simulink model "AC_DC_Converter"  (R2024a)
settings: Solver=VariableStepAuto  StartTime=0.0  StopTime=0.02  RelTol=1e-3
libraries: spsDiodeLib x5, spsSeriesRLCBranchLib x5, spsVoltageMeasurementLib x3, spsACVoltageSourceLib x1, spsLinearTransformerLib x1, spsMosfetLib x1, sps_lib x1
settings Model: Creator=Ketan  LastModifiedBy=Ketan

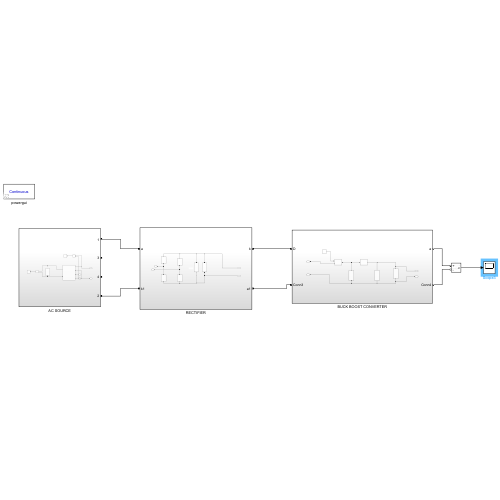
[thumbnail: Simulink's stored preview of the top-level diagram]
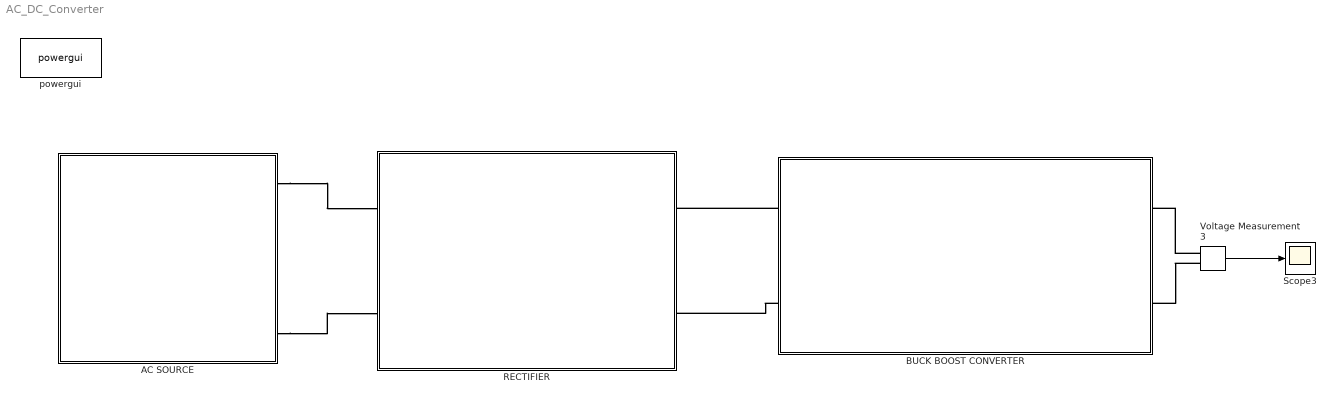
== system AC_DC_Converter ==
  AC SOURCE : Subsystem
  BUCK BOOST CONVERTER : Subsystem
  RECTIFIER : Subsystem
  Scope3 : Scope
  Voltage Measurement3 : spsVoltageMeasurementLib/Voltage Measurement  PhasorSimulation=off  OutputType=Complex  PSBequivalent=0
  powergui : sps_lib/powergui  Priority=1  SimulationMode=Continuous  SampleTime=50e-6  frequency=60  Iterations=50  frequencyindice=50  Pbase=100e6  ErrMax=1e-4  UnitsV=kV  UnitsW=MW  buscounter=0  FunctionMessages=off  echomessages=off  EnableUseOfTLC=off  CurrentSourceSwitches=off  DisableSnubberDevices=off  DisableRonSwitches=off  DisableVfSwitches=off  DisplayEquations=off  AutomaticDiscreteSolvers=off  SolverType=Tustin/Backward Euler (TBE)  Interpol=off  ExternalGateDelay=off  methode=off  Ts=100  x0status=blocks  SPID=on  SwTol=0  HookPort=off  NonlinearTolerance=1e-4  nMaxIteration=100  ContinueOnMaxIteration=off  RestoreLinks=warning  ResistiveCurrentMeasurement=off  Frange=[0:2:500]  Ylog=off  Xlog=on  ShowGrid=off  save=off  variable=ZData  structure=0  ZoomFFT=off  StartTime=0.0  cycles=1  DisplayStyle=1  fundamental=60  FreqAxis=off  MaxFrequency=1000  frequencyindicesteady=1  RmsSteady=1  display=off
  wires:
  Voltage Measurement3/1 -> Scope3/1
  connections:
  BUCK BOOST CONVERTER/LConn1 -- RECTIFIER/RConn1
  Voltage Measurement3/LConn1 -- BUCK BOOST CONVERTER/RConn1
  BUCK BOOST CONVERTER/LConn2 -- RECTIFIER/RConn2
  Voltage Measurement3/LConn2 -- BUCK BOOST CONVERTER/RConn2
  AC SOURCE/RConn1 -- RECTIFIER/LConn1
  AC SOURCE/RConn4 -- RECTIFIER/LConn2

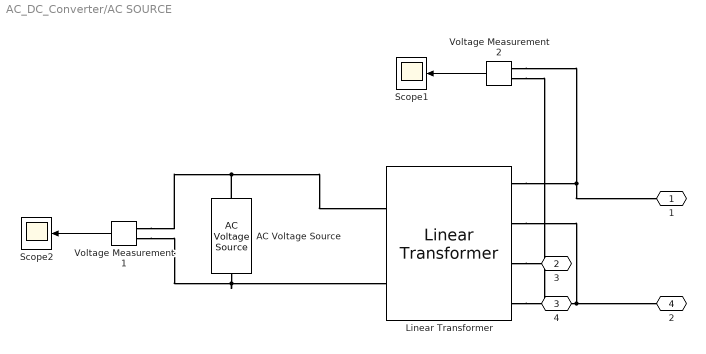
== system AC_DC_Converter/AC SOURCE ==
  AC Voltage Source : spsACVoltageSourceLib/AC Voltage Source  Amplitude=220*sqrt(2)  Phase=0  Frequency=50  SampleTime=0  Measurements=None  BusType=swing  Pref=10e3  Qref=0  Qmin=-inf  Qmax=+inf
  Linear Transformer : spsLinearTransformerLib/Linear Transformer  UNITS=pu  NominalPower=[ 250e6 60 ]  winding1="[ 220  0.002  0.08 ]"  winding2="[ 110  0.002  0.08 ]"  ThreeWindings=on  winding3=[ 110 0.002 0.08 ]  RmLm=[ 500 500 ]  Measurements=None  DataType=off
  Scope1 : Scope
  Scope2 : Scope
  Voltage Measurement1 : spsVoltageMeasurementLib/Voltage Measurement  PhasorSimulation=off  OutputType=Complex  PSBequivalent=0
  Voltage Measurement2 : spsVoltageMeasurementLib/Voltage Measurement  PhasorSimulation=off  OutputType=Complex  PSBequivalent=0
  1 : PMIOPort  Side=Right
  3 : PMIOPort  Port=2  Side=Right
  4 : PMIOPort  Port=3  Side=Right
  2 : PMIOPort  Port=4  Side=Right
  wires:
  Voltage Measurement1/1 -> Scope2/1
  Voltage Measurement2/1 -> Scope1/1
  connections:
  AC Voltage Source/RConn1 -- Linear Transformer/LConn1 -- Voltage Measurement1/LConn1
  AC Voltage Source/LConn1 -- Linear Transformer/LConn2 -- Voltage Measurement1/LConn2
  Voltage Measurement2/LConn2 -- 2/RConn1 -- Linear Transformer/RConn2
  Voltage Measurement2/LConn1 -- 1/RConn1 -- Linear Transformer/RConn1
  Linear Transformer/RConn4 -- 4/RConn1
  Linear Transformer/RConn3 -- 3/RConn1

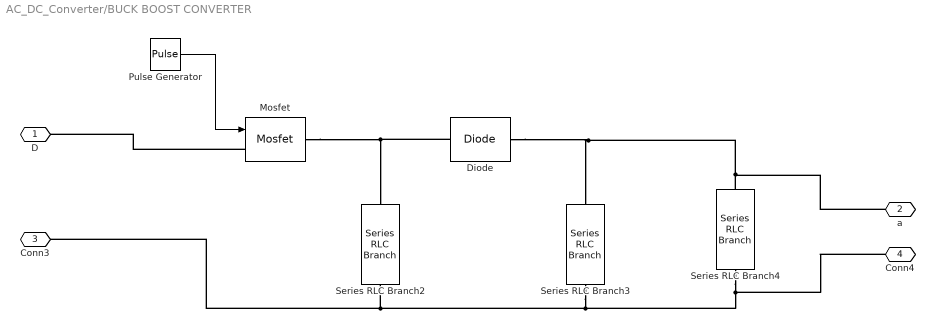
== system AC_DC_Converter/BUCK BOOST CONVERTER ==
  Diode : spsDiodeLib/Diode  Ron=0.001  Lon=0  Vf=0.8  IC=0  UseSnubber=0  Rs=500  Cs=250e-9  Measurements=off
  Mosfet : spsMosfetLib/Mosfet  Ron=0.1  Lon=0  Rd=0.01  Vfd=0  IC=0  Rs=1e5  Cs=inf  Measurements=off
  Pulse Generator : DiscretePulseGenerator  PulseType=Time based  Period=1/40000  PulseWidth=0.536*100
  Series RLC Branch2 : spsSeriesRLCBranchLib/Series RLC Branch  LConnTagsString=__new0  RConnTagsString=__new0  BranchType=L  Resistance=1  Inductance=45e-6  SetiL0=off  InitialCurrent=0  Capacitance=1e-6  Setx0=off  InitialVoltage=0  Measurements=None
  Series RLC Branch3 : spsSeriesRLCBranchLib/Series RLC Branch  LConnTagsString=__new0  RConnTagsString=__new0  BranchType=C  Resistance=1  Inductance=1e-3  SetiL0=off  InitialCurrent=0  Capacitance=8.5e-6  Setx0=off  InitialVoltage=0  Measurements=None
  Series RLC Branch4 : spsSeriesRLCBranchLib/Series RLC Branch  LConnTagsString=__new0  RConnTagsString=__new0  BranchType=R  Resistance=10  Inductance=1e-3  SetiL0=off  InitialCurrent=0  Capacitance=1e-6  Setx0=off  InitialVoltage=0  Measurements=None
  D : PMIOPort  Side=Left
  a : PMIOPort  Port=2  Side=Right
  Conn3 : PMIOPort  Port=3  Side=Left
  Conn4 : PMIOPort  Port=4  Side=Right
  wires:
  Pulse Generator/1 -> Mosfet/1
  connections:
  Mosfet/RConn1 -- Diode/RConn1 -- Series RLC Branch2/LConn1
  Series RLC Branch4/LConn1 -- Diode/LConn1 -- Series RLC Branch3/LConn1 -- a/RConn1
  Mosfet/LConn1 -- D/RConn1
  Series RLC Branch4/RConn1 -- Conn4/RConn1 -- Series RLC Branch3/RConn1 -- Conn3/RConn1 -- Series RLC Branch2/RConn1

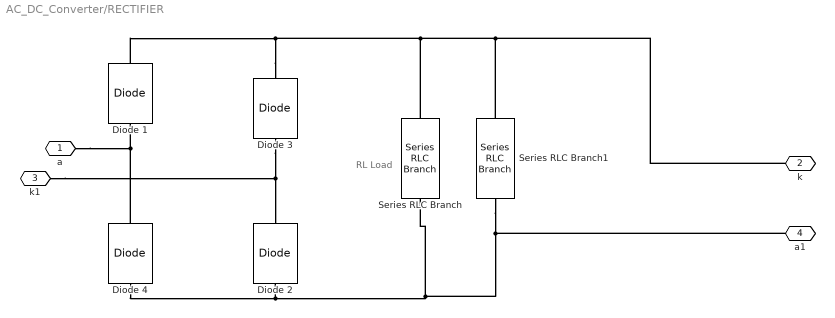
== system AC_DC_Converter/RECTIFIER ==
  note: RL Load
  Diode {1..4} (4 alike) : spsDiodeLib/Diode  Ron=0.001  Lon=0  Vf=0.8  IC=0  UseSnubber=0  Rs=500  Cs=250e-9  Measurements=off
  Series RLC Branch : spsSeriesRLCBranchLib/Series RLC Branch  LConnTagsString=__new0  RConnTagsString=__new0  BranchType=RL  Resistance=1  Inductance=1e-1  SetiL0=off  InitialCurrent=0  Capacitance=0  Setx0=off  InitialVoltage=0  Measurements=None
  Series RLC Branch1 : spsSeriesRLCBranchLib/Series RLC Branch  LConnTagsString=__new0  RConnTagsString=__new0  BranchType=C  Resistance=1  Inductance=1e-1  SetiL0=off  InitialCurrent=0  Capacitance=10e-2  Setx0=off  InitialVoltage=0  Measurements=None
  a : PMIOPort  Side=Left
  k : PMIOPort  Port=2  Side=Right
  k1 : PMIOPort  Port=3  Side=Left
  a1 : PMIOPort  Port=4  Side=Right
  connections:
  Diode 3/LConn1 -- Diode 2/RConn1 -- k1/RConn1
  Diode 3/RConn1 -- k/RConn1 -- Series RLC Branch1/LConn1 -- Series RLC Branch/LConn1 -- Diode 1/RConn1
  Diode 4/RConn1 -- Diode 1/LConn1 -- a/RConn1
  Series RLC Branch1/RConn1 -- Series RLC Branch/RConn1 -- Diode 4/LConn1 -- Diode 2/LConn1 -- a1/RConn1
